simulink model "test_sim_5"  (R2022b)
settings: Solver=ode4  StartTime=0.0  StopTime=10  FixedStep=0.01  RelTol=1e-3
values from neighbouring files (symbols this model uses):
  J = 0.02    [paraset.m]
  Kb = 0.1    [paraset.m]
  Kf = 0.2    [paraset.m]
  Ki = 0.01    [paraset.m]
  Km = 0.1    [paraset.m]
  Kp = 5    [paraset.m]
  L = 0.5    [paraset.m]
  R = 2.0    (= 2)    [paraset.m]
undefined symbols (not defined in the file or in its folder): sigbuilder_block
settings Model: Creator=user  LastModifiedBy=user
settings DataIOCC: ReturnWorkspaceOutputs=off

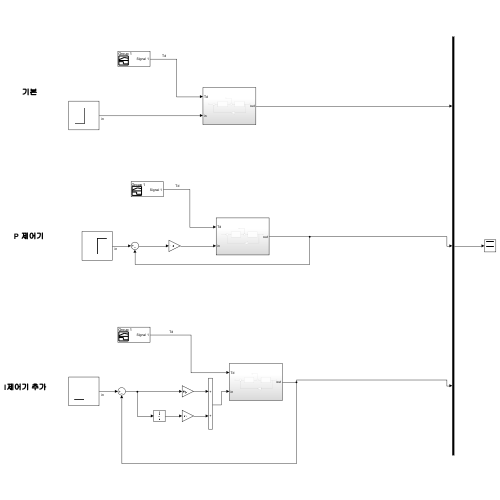
[thumbnail: Simulink's stored preview of the top-level diagram]
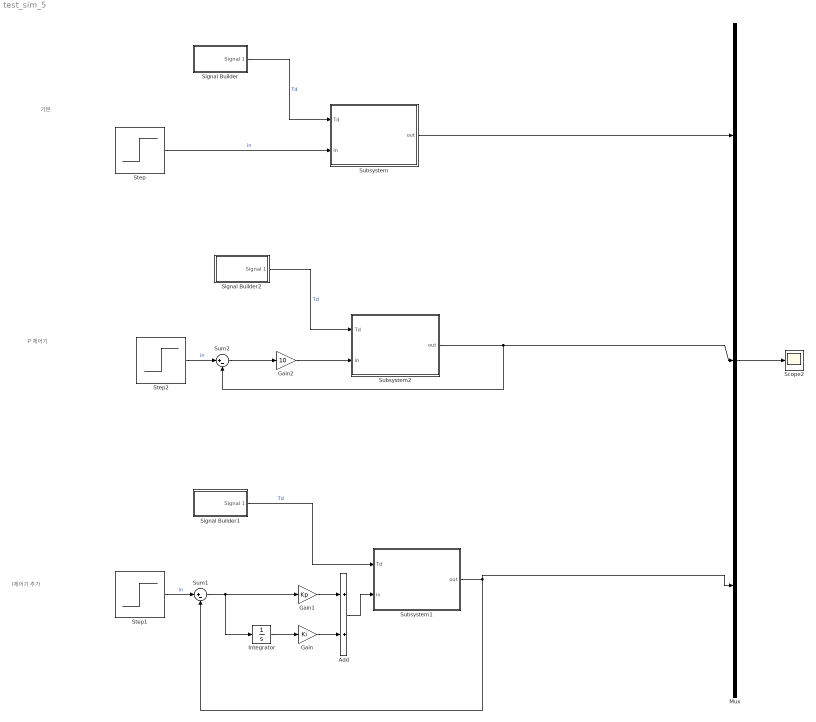
== system test_sim_5 ==
  note: I제어기 추가
  note: 기본
  note: P 제어기
  Add : Sum
  Gain : Gain  Gain=Ki
  Gain1 : Gain  Gain=Kp
  Gain2 : Gain  Gain=10
  Integrator : Integrator
  Mux : Mux  Inputs=3
  Scope2 : Scope
  Signal Builder : Subsystem  Tag=STV Subsys  LoadFcn=sigbuilder_block('load');  StartFcn=sigbuilder_block('start');  StopFcn=sigbuilder_block('stop');  ClipboardFcn=sigbuilder_block('clipboard');  mask(Sigbuilder block){tuvar=[0:10]}
      mask help: Simulink:masks:SigbuilderBlock_MD
      mask init:
      | if ~strcmp(get_param(bdroot(gcbh),'SimulationStatus'),'stopped') tuvar = sigbuilder_block('maskInit'); end
      settings: CopyFcn=sigbuilder_block('copy');  DeleteFcn=sigbuilder_block('delete');  ModelCloseFcn=sigbuilder_block('modelClose');  PreSaveFcn=sigbuilder_block('preSave');  PauseFcn=sigbuilder_block('pause');  ContinueFcn=sigbuilder_block('continue');  NameChangeFcn=sigbuilder_block('namechange');  OpenFcn=sigbuilder_block('open',[626.25 196.5 550.5 399.75 ]);  CloseFcn=sigbuilder_block('close');
      mask Display: plot(0, 0, 100, 100,[2, 2, 32, 32, 2], [68, 8, 8, 68, 68],[32, 2], [38, 38], [32, 19, 2],[53, 60, 44], [32, 17, 17, 2],[16, 16, 31, 31]);txt = getActiveGroup(gcbh);text(2, 100, txt,'verticalAlignment', 'top');
  Signal Builder1 : Subsystem  Tag=STV Subsys  LoadFcn=sigbuilder_block('load');  StartFcn=sigbuilder_block('start');  StopFcn=sigbuilder_block('stop');  ClipboardFcn=sigbuilder_block('clipboard');  mask(Sigbuilder block){tuvar=[0:10]}
      mask help: Simulink:masks:SigbuilderBlock_MD
      mask init:
      | if ~strcmp(get_param(bdroot(gcbh),'SimulationStatus'),'stopped') tuvar = sigbuilder_block('maskInit'); end
      settings: CopyFcn=sigbuilder_block('copy');  DeleteFcn=sigbuilder_block('delete');  ModelCloseFcn=sigbuilder_block('modelClose');  PreSaveFcn=sigbuilder_block('preSave');  PauseFcn=sigbuilder_block('pause');  ContinueFcn=sigbuilder_block('continue');  NameChangeFcn=sigbuilder_block('namechange');  OpenFcn=sigbuilder_block('open',[626.25 196.5 550.5 399.75 ]);  CloseFcn=sigbuilder_block('close');
      mask Display: plot(0, 0, 100, 100,[2, 2, 32, 32, 2], [68, 8, 8, 68, 68],[32, 2], [38, 38], [32, 19, 2],[53, 60, 44], [32, 17, 17, 2],[16, 16, 31, 31]);txt = getActiveGroup(gcbh);text(2, 100, txt,'verticalAlignment', 'top');
  Signal Builder2 : Subsystem  Tag=STV Subsys  LoadFcn=sigbuilder_block('load');  StartFcn=sigbuilder_block('start');  StopFcn=sigbuilder_block('stop');  ClipboardFcn=sigbuilder_block('clipboard');  mask(Sigbuilder block){tuvar=[0:10]}
      mask help: Simulink:masks:SigbuilderBlock_MD
      mask init:
      | if ~strcmp(get_param(bdroot(gcbh),'SimulationStatus'),'stopped') tuvar = sigbuilder_block('maskInit'); end
      settings: CopyFcn=sigbuilder_block('copy');  DeleteFcn=sigbuilder_block('delete');  ModelCloseFcn=sigbuilder_block('modelClose');  PreSaveFcn=sigbuilder_block('preSave');  PauseFcn=sigbuilder_block('pause');  ContinueFcn=sigbuilder_block('continue');  NameChangeFcn=sigbuilder_block('namechange');  OpenFcn=sigbuilder_block('open',[626.25 196.5 550.5 399.75 ]);  CloseFcn=sigbuilder_block('close');
      mask Display: plot(0, 0, 100, 100,[2, 2, 32, 32, 2], [68, 8, 8, 68, 68],[32, 2], [38, 38], [32, 19, 2],[53, 60, 44], [32, 17, 17, 2],[16, 16, 31, 31]);txt = getActiveGroup(gcbh);text(2, 100, txt,'verticalAlignment', 'top');
  Step : Step  After=12  SampleTime=0
  Step1 : Step  After=12  SampleTime=0
  Step2 : Step  After=12  SampleTime=0
  Subsystem : Subsystem
  Subsystem1 : Subsystem
  Subsystem2 : Subsystem
  Sum1 : Sum  Inputs=|+-
  Sum2 : Sum  Inputs=|+-
  wires:
  Signal Builder/1(Signal 1) -> Subsystem/1(Td)  "Td"
  Step/1 -> Subsystem/2(in)  "in"
  Sum1/1 -> Integrator/1, Gain1/1
  Step1/1 -> Sum1/1  "in"
  Subsystem1/1(out) -> Sum1/2, Mux/3
  Signal Builder1/1(Signal 1) -> Subsystem1/1(Td)  "Td"
  Mux/1 -> Scope2/1
  Signal Builder2/1(Signal 1) -> Subsystem2/1(Td)  "Td"
  Subsystem2/1(out) -> Sum2/2, Mux/2
  Step2/1 -> Sum2/1  "in"
  Sum2/1 -> Gain2/1
  Gain2/1 -> Subsystem2/2(in)
  Integrator/1 -> Gain/1
  Gain1/1 -> Add/1
  Gain/1 -> Add/2
  Add/1 -> Subsystem1/2(in)
  Subsystem/1(out) -> Mux/1

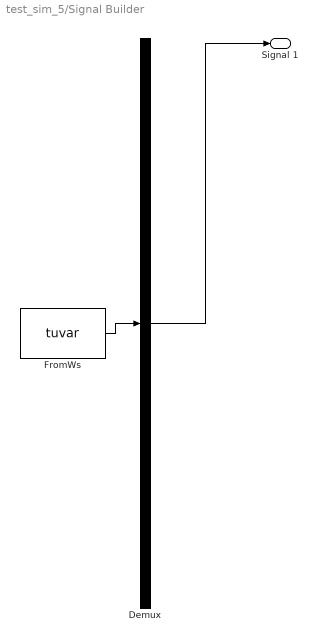
== system test_sim_5/Signal Builder ==
  Demux : Demux  Tag=STV Demux  Outputs=1
      settings: DisplayOption=none
  FromWs : FromWorkspace  Tag=STV FromWs  VariableName=tuvar
      SigBuilderData=|
      | common.afterFinalStr = 'Extrapolate'
      | common.sampleTime = 0
      | dataSet.timeRange = [0 10]
      | dataSet.name = 'Group 1'
      | sbobj.Groups.Name = 'Group 1'
      | sbobj.Groups.Signals.Name = 'Signal 1'
      | sbobj.Groups.Signals.XData = [0 4 4 6 6.04 10]
      | sbobj.Groups.Signals.YData = [0 0 -0.1 -0.1 0 0]
  Signal 1 : Outport  Tag=STV Outport
  wires:
  Demux/1 -> Signal 1/1
  FromWs/1 -> Demux/1

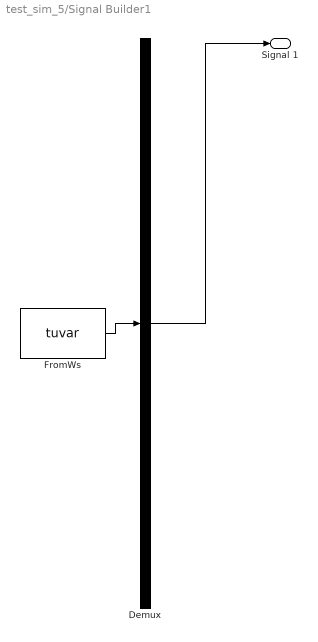
== system test_sim_5/Signal Builder1 ==
  Demux : Demux  Tag=STV Demux  Outputs=1
      settings: DisplayOption=none
  FromWs : FromWorkspace  Tag=STV FromWs  VariableName=tuvar
      SigBuilderData=|
      | common.afterFinalStr = 'Extrapolate'
      | common.sampleTime = 0
      | dataSet.timeRange = [0 10]
      | dataSet.name = 'Group 1'
      | sbobj.Groups.Name = 'Group 1'
      | sbobj.Groups.Signals.Name = 'Signal 1'
      | sbobj.Groups.Signals.XData = [0 4 4 6 6.04 10]
      | sbobj.Groups.Signals.YData = [0 0 -0.1 -0.1 0 0]
  Signal 1 : Outport  Tag=STV Outport
  wires:
  FromWs/1 -> Demux/1
  Demux/1 -> Signal 1/1

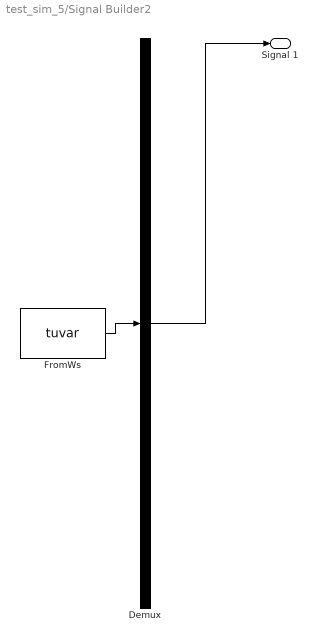
== system test_sim_5/Signal Builder2 ==
  Demux : Demux  Tag=STV Demux  Outputs=1
      settings: DisplayOption=none
  FromWs : FromWorkspace  Tag=STV FromWs  VariableName=tuvar
      SigBuilderData=|
      | common.afterFinalStr = 'Extrapolate'
      | common.sampleTime = 0
      | dataSet.timeRange = [0 10]
      | dataSet.name = 'Group 1'
      | sbobj.Groups.Name = 'Group 1'
      | sbobj.Groups.Signals.Name = 'Signal 1'
      | sbobj.Groups.Signals.XData = [0 4 4 6 6.04 10]
      | sbobj.Groups.Signals.YData = [0 0 -0.1 -0.1 0 0]
  Signal 1 : Outport  Tag=STV Outport
  wires:
  Demux/1 -> Signal 1/1
  FromWs/1 -> Demux/1

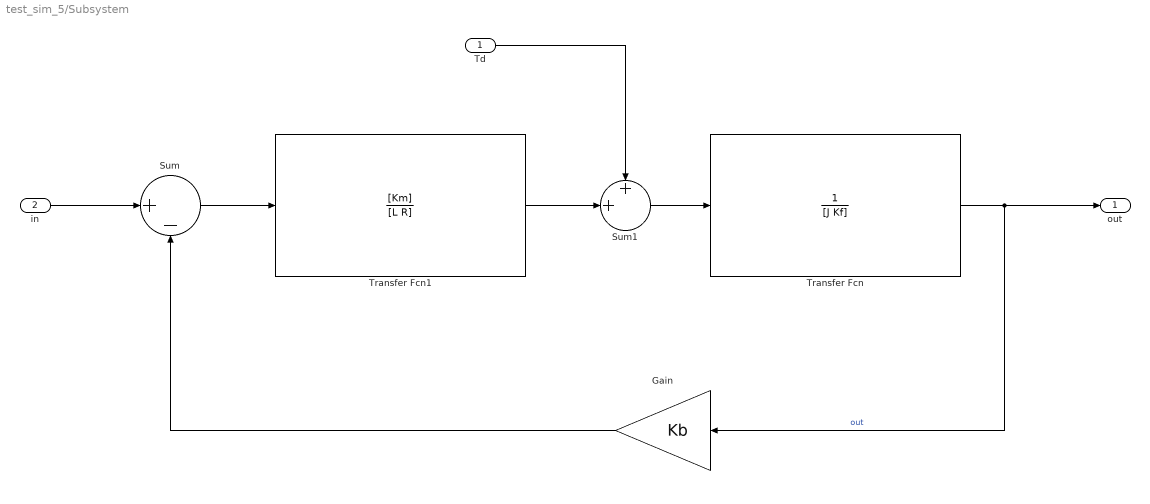
== system test_sim_5/Subsystem ==
  Td : Inport
  in : Inport  Port=2
  Gain : Gain  Gain=Kb
  Sum : Sum  Inputs=|+-
  Sum1 : Sum  Inputs=++|
  Transfer Fcn : TransferFcn  Denominator=[J Kf]
  Transfer Fcn1 : TransferFcn  Numerator=[Km]  Denominator=[L R]
  out : Outport
  wires:
  Transfer Fcn/1 -> out/1, Gain/1  "out"
  Transfer Fcn1/1 -> Sum1/2
  Sum/1 -> Transfer Fcn1/1
  Sum1/1 -> Transfer Fcn/1
  Gain/1 -> Sum/2
  in/1 -> Sum/1
  Td/1 -> Sum1/1

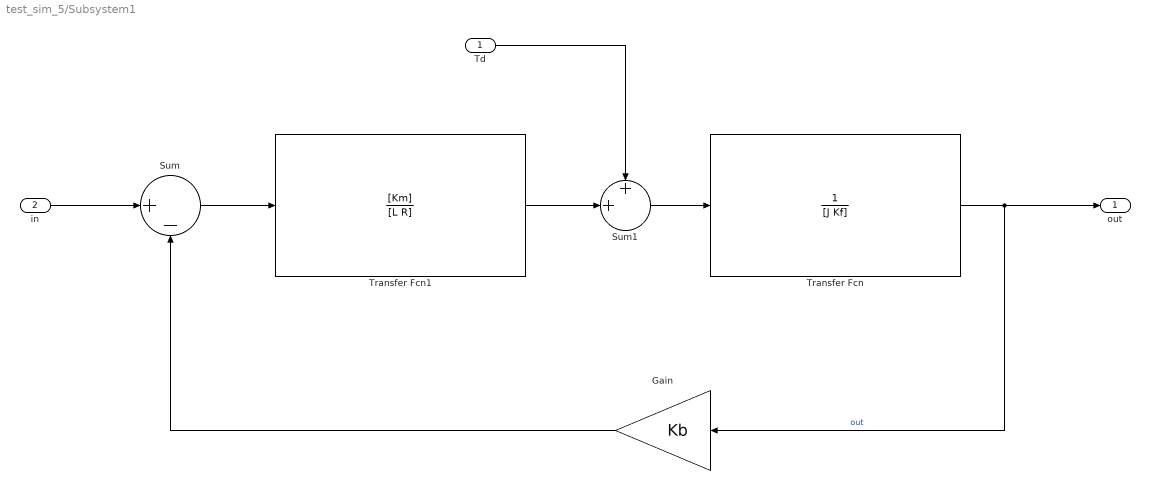
== system test_sim_5/Subsystem1 ==
  Td : Inport
  in : Inport  Port=2
  Gain : Gain  Gain=Kb
  Sum : Sum  Inputs=|+-
  Sum1 : Sum  Inputs=++|
  Transfer Fcn : TransferFcn  Denominator=[J Kf]
  Transfer Fcn1 : TransferFcn  Numerator=[Km]  Denominator=[L R]
  out : Outport
  wires:
  Td/1 -> Sum1/1
  in/1 -> Sum/1
  Gain/1 -> Sum/2
  Sum1/1 -> Transfer Fcn/1
  Sum/1 -> Transfer Fcn1/1
  Transfer Fcn1/1 -> Sum1/2
  Transfer Fcn/1 -> Gain/1, out/1  "out"

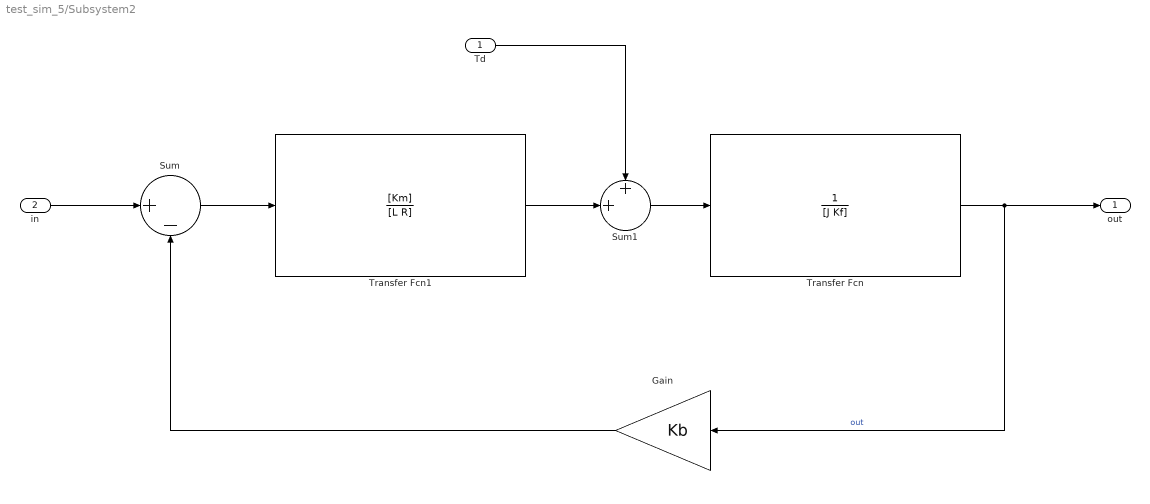
== system test_sim_5/Subsystem2 ==
  Td : Inport
  in : Inport  Port=2
  Gain : Gain  Gain=Kb
  Sum : Sum  Inputs=|+-
  Sum1 : Sum  Inputs=++|
  Transfer Fcn : TransferFcn  Denominator=[J Kf]
  Transfer Fcn1 : TransferFcn  Numerator=[Km]  Denominator=[L R]
  out : Outport
  wires:
  Transfer Fcn/1 -> out/1, Gain/1  "out"
  Transfer Fcn1/1 -> Sum1/2
  Sum/1 -> Transfer Fcn1/1
  Sum1/1 -> Transfer Fcn/1
  Gain/1 -> Sum/2
  in/1 -> Sum/1
  Td/1 -> Sum1/1
